simulink model "dinamica"  (R2022b)
settings: Solver=VariableStepAuto  StartTime=0.0  StopTime=4  RelTol=1e-5
undefined symbols (not defined in the file or in its folder): X, Y, Z
libraries: sm_lib x18, nesl_utility x13
settings Model: Creator=laurc  LastModifiedBy=laurc

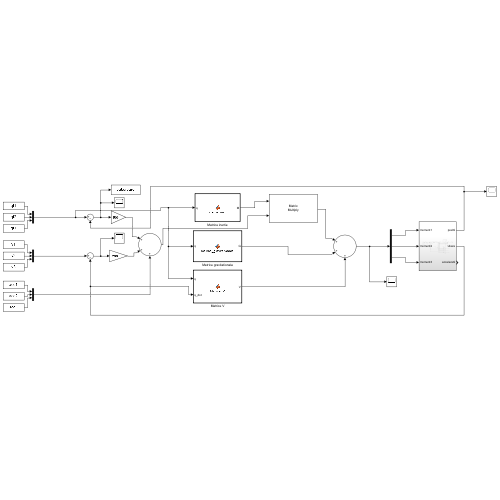
[thumbnail: Simulink's stored preview of the top-level diagram]
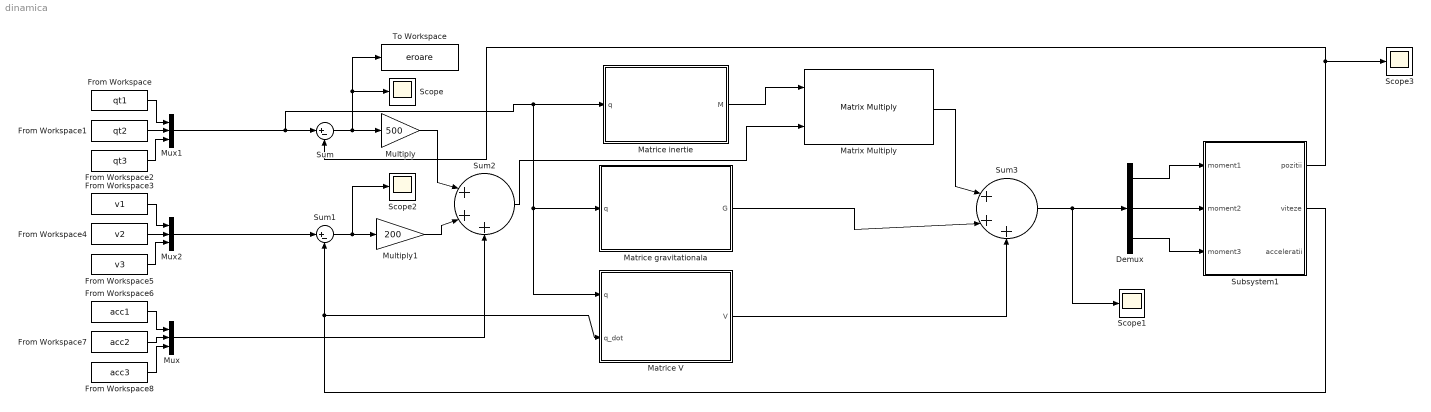
== system dinamica ==
  Demux : Demux  Outputs=3
  From Workspace : FromWorkspace  VariableName=qt1
  From Workspace1 : FromWorkspace  VariableName=qt2
  From Workspace2 : FromWorkspace  VariableName=qt3
  From Workspace3 : FromWorkspace  VariableName=v1
  From Workspace4 : FromWorkspace  VariableName=v2
  From Workspace5 : FromWorkspace  VariableName=v3
  From Workspace6 : FromWorkspace  VariableName=acc1
  From Workspace7 : FromWorkspace  VariableName=acc2
  From Workspace8 : FromWorkspace  VariableName=acc3
  Matrice V : MATLAB Function  TreatAsAtomicUnit=on
  Matrice gravitationala : MATLAB Function  TreatAsAtomicUnit=on
  Matrice inertie : MATLAB Function  TreatAsAtomicUnit=on
  Matrix Multiply : Product  Multiplication=Matrix(*)
  Multiply : Gain  Gain=500
  Multiply1 : Gain  Gain=200
  Mux : Mux  Inputs=3
  Mux1 : Mux  Inputs=3
  Mux2 : Mux  Inputs=3
  Scope{,1..3} (4 alike) : Scope
  Subsystem1 : Subsystem
  Sum : Sum  Inputs=|+-
  Sum1 : Sum  Inputs=|+-
  Sum2 : Sum  Inputs=|+++
  Sum3 : Sum  Inputs=|+++
  To Workspace : ToWorkspace  VariableName=eroare  SaveFormat=Timeseries  SampleTime=-1
  wires:
  Multiply1/1 -> Sum2/2
  Sum/1 -> Scope/1, To Workspace/1, Multiply/1
  From Workspace2/1 -> Mux1/3
  Sum1/1 -> Scope2/1, Multiply1/1
  From Workspace6/1 -> Mux/1
  Multiply/1 -> Sum2/1
  From Workspace7/1 -> Mux/2
  Mux2/1 -> Sum1/1
  Mux/1 -> Sum2/3
  From Workspace5/1 -> Mux2/3
  From Workspace8/1 -> Mux/3
  From Workspace/1 -> Mux1/1
  From Workspace3/1 -> Mux2/1
  From Workspace1/1 -> Mux1/2
  From Workspace4/1 -> Mux2/2
  Matrice inertie/1(M) -> Matrix Multiply/1
  Sum2/1 -> Matrix Multiply/2
  Matrix Multiply/1 -> Sum3/1
  Matrice gravitationala/1(G) -> Sum3/2
  Matrice V/1(V) -> Sum3/3
  Sum3/1 -> Scope1/1, Demux/1
  Demux/1 -> Subsystem1/1(moment1)
  Demux/2 -> Subsystem1/2(moment2)
  Demux/3 -> Subsystem1/3(moment3)
  Subsystem1/1(pozitii) -> Scope3/1, Sum/2
  Subsystem1/2(viteze) -> Sum1/2, Matrice V/2(q_dot)
  Mux1/1 -> Matrice V/1(q), Matrice gravitationala/1(q), Matrice inertie/1(q), Sum/1

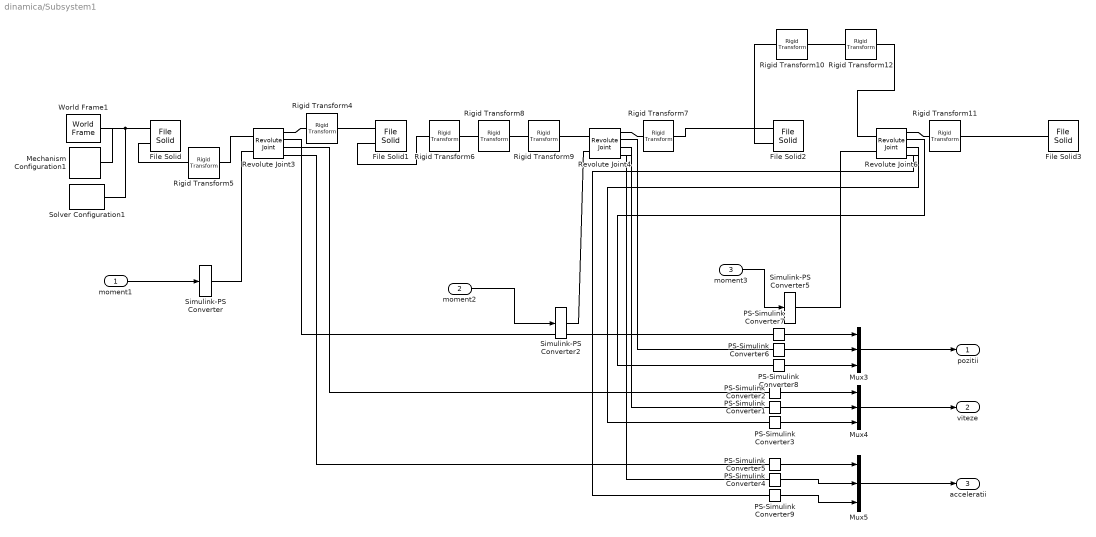
== system dinamica/Subsystem1 ==
  moment1 : Inport
  moment2 : Inport  Port=2
  moment3 : Inport  Port=3
  File Solid : sm_lib/Body Elements/File Solid  ExtGeomFileName=C:\Users\laurc\OneDrive\Desktop\robot puma nou\baza.stp  UnitType=FromFile  ExtGeomFileUnits=m  StepReaderType=HEX  ExportConvexHullGeometry=off  InertiaType=CalculateFromGeometry  Mass=1  MassUnits=kg  CenterOfMass=[0 0 0]  CenterOfMassUnits=m  MomentsOfInertia=[1 1 1]  MomentsOfInertiaUnits=kg*m^2  ProductsOfInertia=[0 0 0]  ProductsOfInertiaUnits=kg*m^2  BasedOnType=Density  Density=1000  DensityUnits=kg/m^3  DoExposeReferenceFrame=on  SerializedFrames=<Frames><Frame><Id>Frame1</Id><Value><Name>F1</Name><Origin><Source>ReferenceFrame</Source><FeatureName></FeatureName></Origin><PrimaryAxis><DefinedDirection>+Z</DefinedDirection><Source>ReferenceFrame</Source><SourceDirection>+Z</SourceDirection><FeatureName></FeatureName></PrimaryAxis><SecondaryAxis><DefinedDirection>+X</DefinedDirection><Source>ReferenceFrame</Source><SourceDirection>+X</SourceDirection><FeatureName></FeatureName></SecondaryAxis></Value></Frame><Frame><Id>Frame2</Id><Value><Name>F2</Name><Origin><Source>GeometricFeature</Source><FeatureName>circular curve 22</FeatureName></Origin><PrimaryAxis><DefinedDirection>+Z</DefinedDirection><Source>ReferenceFrame</Source><SourceDirection>+Z</SourceDirection><FeatureName></FeatureName></PrimaryAxis><SecondaryAxis><DefinedDirection>+X</DefinedDirection><Source>ReferenceFrame</Source><SourceDirection>+X</SourceDirection><FeatureName></FeatureName></SecondaryAxis></Value></Frame></Frames>  GraphicType=FromGeometry  MarkerShape=Sphere  MarkerSize=10  GraphicVisPropType=SimpleVisualProperties  GraphicDiffuseColor=[0.8 0.8 0.8]  GraphicSpecularColor=[0.5 0.5 0.5 1.0]  GraphicAmbientColor=[0.15 0.15 0.15 1.0]  GraphicEmissiveColor=[0.0 0.0 0.0 1.0]  GraphicShininess=75  GraphicOpacity=1.0
  File Solid1 : sm_lib/Body Elements/File Solid  ExtGeomFileName=C:\Users\laurc\OneDrive\Desktop\robot puma nou\brat1.stp  UnitType=FromFile  ExtGeomFileUnits=m  StepReaderType=HEX  ExportConvexHullGeometry=off  InertiaType=CalculateFromGeometry  Mass=1  MassUnits=kg  CenterOfMass=[0 0 0]  CenterOfMassUnits=m  MomentsOfInertia=[1 1 1]  MomentsOfInertiaUnits=kg*m^2  ProductsOfInertia=[0 0 0]  ProductsOfInertiaUnits=kg*m^2  BasedOnType=Density  Density=1000  DensityUnits=kg/m^3  DoExposeReferenceFrame=on  SerializedFrames=<Frames><Frame><Id>Frame1</Id><Value><Name>F1</Name><Origin><Source>GeometricFeature</Source><FeatureName>planar surface 1</FeatureName></Origin><PrimaryAxis><DefinedDirection>+Z</DefinedDirection><Source>ReferenceFrame</Source><SourceDirection>+Z</SourceDirection><FeatureName></FeatureName></PrimaryAxis><SecondaryAxis><DefinedDirection>+X</DefinedDirection><Source>ReferenceFrame</Source><SourceDirection>+X</SourceDirection><FeatureName></FeatureName></SecondaryAxis></Value></Frame><Frame><Id>Frame2</Id><Value><Name>F2</Name><Origin><Source>GeometricFeature</Source><FeatureName>planar surface 3</FeatureName></Origin><PrimaryAxis><DefinedDirection>+Z</DefinedDirection><Source>ReferenceFrame</Source><SourceDirection>+Z</SourceDirection><FeatureName></FeatureName></PrimaryAxis><SecondaryAxis><DefinedDirection>+X</DefinedDirection><Source>ReferenceFrame</Source><SourceDirection>+X</SourceDirection><FeatureName></FeatureName></SecondaryAxis></Value></Frame></Frames>  GraphicType=FromGeometry  MarkerShape=Sphere  MarkerSize=10  GraphicVisPropType=SimpleVisualProperties  GraphicDiffuseColor=[0.8 0.8 0.8]  GraphicSpecularColor=[0.5 0.5 0.5 1.0]  GraphicAmbientColor=[0.15 0.15 0.15 1.0]  GraphicEmissiveColor=[0.0 0.0 0.0 1.0]  GraphicShininess=75  GraphicOpacity=1.0
  File Solid2 : sm_lib/Body Elements/File Solid  ExtGeomFileName=C:\Users\laurc\OneDrive\Desktop\robot puma nou\brat2.stp  UnitType=FromFile  ExtGeomFileUnits=m  StepReaderType=HEX  ExportConvexHullGeometry=off  InertiaType=CalculateFromGeometry  Mass=1  MassUnits=kg  CenterOfMass=[0 0 0]  CenterOfMassUnits=m  MomentsOfInertia=[1 1 1]  MomentsOfInertiaUnits=kg*m^2  ProductsOfInertia=[0 0 0]  ProductsOfInertiaUnits=kg*m^2  BasedOnType=Density  Density=1000  DensityUnits=kg/m^3  DoExposeReferenceFrame=on  SerializedFrames=<Frames><Frame><Id>Frame1</Id><Value><Name>F1</Name><Origin><Source>GeometricFeature</Source><FeatureName>planar surface 2</FeatureName></Origin><PrimaryAxis><DefinedDirection>+X</DefinedDirection><Source>ReferenceFrame</Source><SourceDirection>+Z</SourceDirection><FeatureName></FeatureName></PrimaryAxis><SecondaryAxis><DefinedDirection>-Y</DefinedDirection><Source>ReferenceFrame</Source><SourceDirection>+X</SourceDirection><FeatureName></FeatureName></SecondaryAxis></Value></Frame><Frame><Id>Frame2</Id><Value><Name>F2</Name><Origin><Source>GeometricFeature</Source><FeatureName>planar surface 1</FeatureName></Origin><PrimaryAxis><DefinedDirection>+Z</DefinedDirection><Source>ReferenceFrame</Source><SourceDirection>+Z</SourceDirection><FeatureName></FeatureName></PrimaryAxis><SecondaryAxis><DefinedDirection>+X</DefinedDirection><Source>ReferenceFrame</Source><SourceDirection>+X</SourceDirection><FeatureName></FeatureName></SecondaryAxis></Value></Frame></Frames>  GraphicType=FromGeometry  MarkerShape=Sphere  MarkerSize=10  GraphicVisPropType=SimpleVisualProperties  GraphicDiffuseColor=[0.8 0.8 0.8]  GraphicSpecularColor=[0.5 0.5 0.5 1.0]  GraphicAmbientColor=[0.15 0.15 0.15 1.0]  GraphicEmissiveColor=[0.0 0.0 0.0 1.0]  GraphicShininess=75  GraphicOpacity=1.0
  File Solid3 : sm_lib/Body Elements/File Solid  ExtGeomFileName=C:\Users\laurc\OneDrive\Desktop\robot puma nou\efector.stp  UnitType=FromFile  ExtGeomFileUnits=m  StepReaderType=HEX  ExportConvexHullGeometry=off  InertiaType=CalculateFromGeometry  Mass=1  MassUnits=kg  CenterOfMass=[0 0 0]  CenterOfMassUnits=m  MomentsOfInertia=[1 1 1]  MomentsOfInertiaUnits=kg*m^2  ProductsOfInertia=[0 0 0]  ProductsOfInertiaUnits=kg*m^2  BasedOnType=Density  Density=1000  DensityUnits=kg/m^3  DoExposeReferenceFrame=on  SerializedFrames=<Frames><Frame><Id>Frame1</Id><Value><Name>F1</Name><Origin><Source>GeometricFeature</Source><FeatureName>planar surface 12</FeatureName></Origin><PrimaryAxis><DefinedDirection>+Z</DefinedDirection><Source>ReferenceFrame</Source><SourceDirection>+Z</SourceDirection><FeatureName></FeatureName></PrimaryAxis><SecondaryAxis><DefinedDirection>+X</DefinedDirection><Source>ReferenceFrame</Source><SourceDirection>+X</SourceDirection><FeatureName></FeatureName></SecondaryAxis></Value></Frame></Frames>  GraphicType=FromGeometry  MarkerShape=Sphere  MarkerSize=10  GraphicVisPropType=SimpleVisualProperties  GraphicDiffuseColor=[0.8 0.8 0.8]  GraphicSpecularColor=[0.5 0.5 0.5 1.0]  GraphicAmbientColor=[0.15 0.15 0.15 1.0]  GraphicEmissiveColor=[0.0 0.0 0.0 1.0]  GraphicShininess=75  GraphicOpacity=1.0
  Mechanism Configuration1 : sm_lib/Utilities/Mechanism Configuration  UniformGravity=Constant  GravityVector=[0 0 -9.80665]  GravityUnits=m/s^2  LinearizationDelta=0.001  JointModeTransitionNonlinearIterations=2
  Mux3 : Mux  Inputs=3
  Mux4 : Mux  Inputs=3
  Mux5 : Mux  Inputs=3
  PS-Simulink Converter{1..9} (9 alike) : nesl_utility/PS-Simulink Converter  PhysicalDomain=network_engine_domain  SubClassName=ps_output  LeftPortType=input  RightPortType=output  PseudoPeriodic=off  Frequencies=[]  VectorFormat=inherit  Unit=inherit  AffineConversion=off
  Revolute Joint3 : sm_lib/Joints/Revolute Joint  JointMode=Normal  SenseConstraintForce=off  SenseConstraintForceX=off  SenseConstraintForceY=off  SenseConstraintForceZ=off  SenseConstraintTorque=off  SenseConstraintTorqueX=off  SenseConstraintTorqueY=off  SenseConstraintTorqueZ=off  SenseTotalForce=off  SenseTotalForceX=off  SenseTotalForceY=off  SenseTotalForceZ=off  SenseTotalTorque=off  SenseTotalTorqueX=off  SenseTotalTorqueY=off  SenseTotalTorqueZ=off  CompositeWrenchDir=FollowerOnBase  CompositeWrenchFrame=BaseFrame  EquilibriumPosition=0  EquilibriumPositionUnits=deg  SpringStiffness=0  SpringStiffnessUnits=N*m/deg  DampingCoefficient=0  DampingCoefficientUnits=N*m/(deg/s)  TorqueActuationMode=ComputedTorque  MotionActuationMode=InputMotion  SensePosition=on  SenseVelocity=on  SenseAcceleration=on  SenseTorqueForce=off  SenseLowerLimitTorqueForce=off  SenseUpperLimitTorqueForce=off  LowerLimitSpecify=off  LowerLimitBound=-90  LowerLimitBoundUnits=deg  LowerLimitStiffness=1e4  LowerLimitStiffnessUnits=N*m/deg  LowerLimitDamping=10  LowerLimitDampingUnits=N*m/(deg/s)  LowerLimitTransitionRegionWidth=0.1  LowerLimitTransitionRegionWidthUnits=deg  UpperLimitSpecify=off  UpperLimitBound=90  UpperLimitBoundUnits=deg  UpperLimitStiffness=1e4  UpperLimitStiffnessUnits=N*m/deg  UpperLimitDamping=10  UpperLimitDampingUnits=N*m/(deg/s)  UpperLimitTransitionRegionWidth=0.1  UpperLimitTransitionRegionWidthUnits=deg  PositionTargetSpecify=off  PositionTargetPriority=High  PositionTargetValue=0  PositionTargetValueUnits=deg  VelocityTargetSpecify=off  VelocityTargetPriority=High  VelocityTargetValue=0  VelocityTargetValueUnits=deg/s
  Revolute Joint4 : sm_lib/Joints/Revolute Joint  JointMode=Normal  SenseConstraintForce=off  SenseConstraintForceX=off  SenseConstraintForceY=off  SenseConstraintForceZ=off  SenseConstraintTorque=off  SenseConstraintTorqueX=off  SenseConstraintTorqueY=off  SenseConstraintTorqueZ=off  SenseTotalForce=off  SenseTotalForceX=off  SenseTotalForceY=off  SenseTotalForceZ=off  SenseTotalTorque=off  SenseTotalTorqueX=off  SenseTotalTorqueY=off  SenseTotalTorqueZ=off  CompositeWrenchDir=FollowerOnBase  CompositeWrenchFrame=BaseFrame  EquilibriumPosition=0  EquilibriumPositionUnits=deg  SpringStiffness=0  SpringStiffnessUnits=N*m/deg  DampingCoefficient=0  DampingCoefficientUnits=N*m/(deg/s)  TorqueActuationMode=ComputedTorque  MotionActuationMode=InputMotion  SensePosition=on  SenseVelocity=on  SenseAcceleration=on  SenseTorqueForce=off  SenseLowerLimitTorqueForce=off  SenseUpperLimitTorqueForce=off  LowerLimitSpecify=off  LowerLimitBound=-90  LowerLimitBoundUnits=deg  LowerLimitStiffness=1e4  LowerLimitStiffnessUnits=N*m/deg  LowerLimitDamping=10  LowerLimitDampingUnits=N*m/(deg/s)  LowerLimitTransitionRegionWidth=0.1  LowerLimitTransitionRegionWidthUnits=deg  UpperLimitSpecify=off  UpperLimitBound=90  UpperLimitBoundUnits=deg  UpperLimitStiffness=1e4  UpperLimitStiffnessUnits=N*m/deg  UpperLimitDamping=10  UpperLimitDampingUnits=N*m/(deg/s)  UpperLimitTransitionRegionWidth=0.1  UpperLimitTransitionRegionWidthUnits=deg  PositionTargetSpecify=off  PositionTargetPriority=High  PositionTargetValue=0  PositionTargetValueUnits=deg  VelocityTargetSpecify=off  VelocityTargetPriority=High  VelocityTargetValue=0  VelocityTargetValueUnits=deg/s
  Revolute Joint6 : sm_lib/Joints/Revolute Joint  JointMode=Normal  SenseConstraintForce=off  SenseConstraintForceX=off  SenseConstraintForceY=off  SenseConstraintForceZ=off  SenseConstraintTorque=off  SenseConstraintTorqueX=off  SenseConstraintTorqueY=off  SenseConstraintTorqueZ=off  SenseTotalForce=off  SenseTotalForceX=off  SenseTotalForceY=off  SenseTotalForceZ=off  SenseTotalTorque=off  SenseTotalTorqueX=off  SenseTotalTorqueY=off  SenseTotalTorqueZ=off  CompositeWrenchDir=FollowerOnBase  CompositeWrenchFrame=BaseFrame  EquilibriumPosition=0  EquilibriumPositionUnits=deg  SpringStiffness=0  SpringStiffnessUnits=N*m/deg  DampingCoefficient=0  DampingCoefficientUnits=N*m/(deg/s)  TorqueActuationMode=ComputedTorque  MotionActuationMode=InputMotion  SensePosition=on  SenseVelocity=on  SenseAcceleration=on  SenseTorqueForce=off  SenseLowerLimitTorqueForce=off  SenseUpperLimitTorqueForce=off  LowerLimitSpecify=off  LowerLimitBound=-90  LowerLimitBoundUnits=deg  LowerLimitStiffness=1e4  LowerLimitStiffnessUnits=N*m/deg  LowerLimitDamping=10  LowerLimitDampingUnits=N*m/(deg/s)  LowerLimitTransitionRegionWidth=0.1  LowerLimitTransitionRegionWidthUnits=deg  UpperLimitSpecify=off  UpperLimitBound=90  UpperLimitBoundUnits=deg  UpperLimitStiffness=1e4  UpperLimitStiffnessUnits=N*m/deg  UpperLimitDamping=10  UpperLimitDampingUnits=N*m/(deg/s)  UpperLimitTransitionRegionWidth=0.1  UpperLimitTransitionRegionWidthUnits=deg  PositionTargetSpecify=off  PositionTargetPriority=High  PositionTargetValue=0  PositionTargetValueUnits=deg  VelocityTargetSpecify=off  VelocityTargetPriority=High  VelocityTargetValue=0  VelocityTargetValueUnits=deg/s
  Rigid Transform10 : sm_lib/Frames and Transforms/Rigid Transform  TranslationMethod=Cartesian  TranslationStandardOffset=0  TranslationLengthUnit=mm  TranslationStandardAxis=+Z  TranslationCartesianOffset=[0 -0 -60]  TranslationROffset=0  TranslationROffsetUnits=m  TranslationZOffset=0  TranslationZOffsetUnits=m  TranslationThetaOffset=0  TranslationThetaOffsetUnits=deg  RotationMethod=StandardAxis  RotationAngleUnits=deg  RotationStandardAxis=-Y  RotationAngle=90  RotationArbitraryAxis=[0 0 1]  FollAlignAxisA=+X  BaseAlignAxisA=+Y  FollAlignAxisB=+Y  BaseAlignAxisB=+Z  RotationSequenceAxes=FollowerAxes  RotationSequence=XYX  RotationSequenceAngles=[0 0 0]  RotationSequenceAnglesUnits=deg  RotationMatrix=[1 0 0; 0 1 0; 0 0 1]  Quaternion=[1 0 0 0]
  Rigid Transform11 : sm_lib/Frames and Transforms/Rigid Transform  TranslationMethod=Cartesian  TranslationStandardOffset=0  TranslationLengthUnit=mm  TranslationStandardAxis=+Z  TranslationCartesianOffset=[0 0 0]  TranslationROffset=0  TranslationROffsetUnits=m  TranslationZOffset=0  TranslationZOffsetUnits=m  TranslationThetaOffset=0  TranslationThetaOffsetUnits=deg  RotationMethod=StandardAxis  RotationAngleUnits=deg  RotationStandardAxis=+Y  RotationAngle=90  RotationArbitraryAxis=[0 0 1]  FollAlignAxisA=+X  BaseAlignAxisA=+Y  FollAlignAxisB=+Y  BaseAlignAxisB=+Z  RotationSequenceAxes=FollowerAxes  RotationSequence=XYX  RotationSequenceAngles=[0 0 0]  RotationSequenceAnglesUnits=deg  RotationMatrix=[1 0 0; 0 1 0; 0 0 1]  Quaternion=[1 0 0 0]
  Rigid Transform12 : sm_lib/Frames and Transforms/Rigid Transform  TranslationMethod=Cartesian  TranslationStandardOffset=0  TranslationLengthUnit=mm  TranslationStandardAxis=+Z  TranslationCartesianOffset=[0 0 0]  TranslationROffset=0  TranslationROffsetUnits=m  TranslationZOffset=0  TranslationZOffsetUnits=m  TranslationThetaOffset=0  TranslationThetaOffsetUnits=deg  RotationMethod=StandardAxis  RotationAngleUnits=deg  RotationStandardAxis=-Y  RotationAngle=90  RotationArbitraryAxis=[0 0 1]  FollAlignAxisA=+X  BaseAlignAxisA=+Y  FollAlignAxisB=+Y  BaseAlignAxisB=+Z  RotationSequenceAxes=FollowerAxes  RotationSequence=XYX  RotationSequenceAngles=[0 0 0]  RotationSequenceAnglesUnits=deg  RotationMatrix=[1 0 0; 0 1 0; 0 0 1]  Quaternion=[1 0 0 0]
  Rigid Transform4 : sm_lib/Frames and Transforms/Rigid Transform  TranslationMethod=None  TranslationStandardOffset=0  TranslationLengthUnit=mm  TranslationStandardAxis=+Z  TranslationCartesianOffset=0  TranslationROffset=0  TranslationROffsetUnits=m  TranslationZOffset=0  TranslationZOffsetUnits=m  TranslationThetaOffset=0  TranslationThetaOffsetUnits=deg  RotationMethod=StandardAxis  RotationAngleUnits=deg  RotationStandardAxis=-Y  RotationAngle=90  RotationArbitraryAxis=[0 0 1]  FollAlignAxisA=+X  BaseAlignAxisA=+Y  FollAlignAxisB=+Y  BaseAlignAxisB=+Z  RotationSequenceAxes=FollowerAxes  RotationSequence=XYX  RotationSequenceAngles=[0 0 0]  RotationSequenceAnglesUnits=deg  RotationMatrix=[1 0 0; 0 1 0; 0 0 1]  Quaternion=[1 0 0 0]
  Rigid Transform5 : sm_lib/Frames and Transforms/Rigid Transform  TranslationMethod=Cartesian  TranslationStandardOffset=0  TranslationLengthUnit=mm  TranslationStandardAxis=+Y  TranslationCartesianOffset=[0 31 0]  TranslationROffset=0  TranslationROffsetUnits=m  TranslationZOffset=0  TranslationZOffsetUnits=m  TranslationThetaOffset=0  TranslationThetaOffsetUnits=deg  RotationMethod=StandardAxis  RotationAngleUnits=deg  RotationStandardAxis=+X  RotationAngle=90  RotationArbitraryAxis=[0 0 1]  FollAlignAxisA=+X  BaseAlignAxisA=+Y  FollAlignAxisB=+Y  BaseAlignAxisB=+Z  RotationSequenceAxes=FollowerAxes  RotationSequence=XYX  RotationSequenceAngles=[0 0 0]  RotationSequenceAnglesUnits=deg  RotationMatrix=[1 0 0; 0 1 0; 0 0 1]  Quaternion=[1 0 0 0]
  Rigid Transform6 : sm_lib/Frames and Transforms/Rigid Transform  TranslationMethod=Cartesian  TranslationStandardOffset=0  TranslationLengthUnit=mm  TranslationStandardAxis=+Z  TranslationCartesianOffset=[0 30 0]  TranslationROffset=0  TranslationROffsetUnits=m  TranslationZOffset=0  TranslationZOffsetUnits=m  TranslationThetaOffset=0  TranslationThetaOffsetUnits=deg  RotationMethod=StandardAxis  RotationAngleUnits=deg  RotationStandardAxis=-X  RotationAngle=90  RotationArbitraryAxis=[0 0 1]  FollAlignAxisA=+X  BaseAlignAxisA=+Y  FollAlignAxisB=+Y  BaseAlignAxisB=+Z  RotationSequenceAxes=FollowerAxes  RotationSequence=XYX  RotationSequenceAngles=[0 0 0]  RotationSequenceAnglesUnits=deg  RotationMatrix=[1 0 0; 0 1 0; 0 0 1]  Quaternion=[1 0 0 0]
  Rigid Transform7 : sm_lib/Frames and Transforms/Rigid Transform  TranslationMethod=None  TranslationStandardOffset=0  TranslationLengthUnit=mm  TranslationStandardAxis=+Z  TranslationCartesianOffset=[0 294.5 141.5]  TranslationROffset=0  TranslationROffsetUnits=m  TranslationZOffset=0  TranslationZOffsetUnits=m  TranslationThetaOffset=0  TranslationThetaOffsetUnits=deg  RotationMethod=StandardAxis  RotationAngleUnits=deg  RotationStandardAxis=+Y  RotationAngle=90  RotationArbitraryAxis=[0 0 1]  FollAlignAxisA=+X  BaseAlignAxisA=+Y  FollAlignAxisB=+Y  BaseAlignAxisB=+Z  RotationSequenceAxes=FollowerAxes  RotationSequence=XYX  RotationSequenceAngles=[0 0 0]  RotationSequenceAnglesUnits=deg  RotationMatrix=[1 0 0; 0 1 0; 0 0 1]  Quaternion=[1 0 0 0]
  Rigid Transform8 : sm_lib/Frames and Transforms/Rigid Transform  TranslationMethod=Cartesian  TranslationStandardOffset=0  TranslationLengthUnit=mm  TranslationStandardAxis=+Z  TranslationCartesianOffset=[0 0 30]  TranslationROffset=0  TranslationROffsetUnits=m  TranslationZOffset=0  TranslationZOffsetUnits=m  TranslationThetaOffset=0  TranslationThetaOffsetUnits=deg  RotationMethod=StandardAxis  RotationAngleUnits=deg  RotationStandardAxis=-Y  RotationAngle=90  RotationArbitraryAxis=[0 0 1]  FollAlignAxisA=+X  BaseAlignAxisA=+Y  FollAlignAxisB=+Y  BaseAlignAxisB=+Z  RotationSequenceAxes=FollowerAxes  RotationSequence=XYX  RotationSequenceAngles=[0 0 0]  RotationSequenceAnglesUnits=deg  RotationMatrix=[1 0 0; 0 1 0; 0 0 1]  Quaternion=[1 0 0 0]
  Rigid Transform9 : sm_lib/Frames and Transforms/Rigid Transform  TranslationMethod=None  TranslationStandardOffset=0  TranslationLengthUnit=mm  TranslationStandardAxis=+Z  TranslationCartesianOffset=[0 294.5 141.5]  TranslationROffset=0  TranslationROffsetUnits=m  TranslationZOffset=0  TranslationZOffsetUnits=m  TranslationThetaOffset=0  TranslationThetaOffsetUnits=deg  RotationMethod=StandardAxis  RotationAngleUnits=deg  RotationStandardAxis=+Y  RotationAngle=90  RotationArbitraryAxis=[0 0 1]  FollAlignAxisA=+X  BaseAlignAxisA=+Y  FollAlignAxisB=+Y  BaseAlignAxisB=+Z  RotationSequenceAxes=FollowerAxes  RotationSequence=XYX  RotationSequenceAngles=[0 0 0]  RotationSequenceAnglesUnits=deg  RotationMatrix=[1 0 0; 0 1 0; 0 0 1]  Quaternion=[1 0 0 0]
  Simulink-PS Converter : nesl_utility/Simulink-PS Converter  PhysicalDomain=network_engine_domain  SubClassName=ps_input  LeftPortType=input  RightPortType=output  PseudoPeriodic=off  Frequencies=[]  NoiseDistribution=none  NoiseParameters=[]  Unit=1  AffineConversion=off  FilteringAndDerivatives=filter  SimscapeFilterOrder=2  InputFilterTimeConstant=0.001  UdotUserProvided=0
  Simulink-PS Converter2 : nesl_utility/Simulink-PS Converter  PhysicalDomain=network_engine_domain  SubClassName=ps_input  LeftPortType=input  RightPortType=output  PseudoPeriodic=off  Frequencies=[]  NoiseDistribution=none  NoiseParameters=[]  Unit=1  AffineConversion=off  FilteringAndDerivatives=filter  SimscapeFilterOrder=2  InputFilterTimeConstant=0.001  UdotUserProvided=0
  Simulink-PS Converter5 : nesl_utility/Simulink-PS Converter  PhysicalDomain=network_engine_domain  SubClassName=ps_input  LeftPortType=input  RightPortType=output  PseudoPeriodic=off  Frequencies=[]  NoiseDistribution=none  NoiseParameters=[]  Unit=1  AffineConversion=off  FilteringAndDerivatives=filter  SimscapeFilterOrder=2  InputFilterTimeConstant=0.001  UdotUserProvided=0
  Solver Configuration1 : nesl_utility/Solver Configuration  PhysicalDomain=network_engine_domain  SubClassName=solver  LeftPortType=input  RightPortType=generic  Tones=[]  Harmonics=[]  SimulateNoise=off  Profile=off  UseLocalSampling=off  EnableSwitchedLinearOptims=on  FrequencyDomain=off  UseCCode=off  RelTol=0.001  AbsTol=0.001  MinStep=1e-09  ToWorkspace=off  RevertToSquareIcSolve=off  NumHomotopyIterations=100  PhasorMode=off  PhasorModeNumHarmonics=1  ConsistencySolver=NEWTON_XTOL_AFTER_FTOL  IndexReductionMethod=DerivativeReplacement  DoDC=off  ResidualTolerance=1e-09  ConsistencyTolSource=GLOBAL  ConsistencyAbsTol=0.001  ConsistencyRelTol=0.001  ConsistencyTolFactor=0.001  UseLocalSolver=off  LocalSolverChoice=NE_BACKWARD_EULER_ADVANCER  ResolveIndetEquations=on  FunctionEvalNumThread=1  LocalSolverSampleTime=0.001  DoFixedCost=off  MaxNonlinIter=3  MaxModeIter=2  ComputeImpulses=off  ImpulseIterations=2  LinearAlgebra=auto  LinearAlgebraNumThread=0  EquationFormulation=NE_TIME_EF  DelaysMemoryBudget=1024  AutomaticFiltering=on  FilteringTimeConstant=0.001  PartitionStorageMethod=AS_NEEDED  PartitionMemoryBudget=1024  PartitionMethod=ROBUST
  World Frame1 : sm_lib/Frames and Transforms/World Frame
  pozitii : Outport
  viteze : Outport  Port=2
  acceleratii : Outport  Port=3
  wires:
  Mux4/1 -> viteze/1
  moment2/1 -> Simulink-PS Converter2/1
  moment3/1 -> Simulink-PS Converter5/1
  PS-Simulink Converter4/1 -> Mux5/2
  Mux5/1 -> acceleratii/1
  PS-Simulink Converter7/1 -> Mux3/1
  PS-Simulink Converter2/1 -> Mux4/1
  PS-Simulink Converter8/1 -> Mux3/3
  PS-Simulink Converter1/1 -> Mux4/2
  Mux3/1 -> pozitii/1
  PS-Simulink Converter9/1 -> Mux5/3
  PS-Simulink Converter3/1 -> Mux4/3
  PS-Simulink Converter5/1 -> Mux5/1
  moment1/1 -> Simulink-PS Converter/1
  PS-Simulink Converter6/1 -> Mux3/2
  connections:
  Revolute Joint4/RConn3 -- PS-Simulink Converter1/LConn1
  Revolute Joint4/RConn2 -- PS-Simulink Converter6/LConn1
  Rigid Transform7/RConn1 -- File Solid2/LConn1
  Rigid Transform6/RConn1 -- Rigid Transform8/LConn1
  Revolute Joint6/RConn3 -- PS-Simulink Converter3/LConn1
  Revolute Joint6/RConn1 -- Rigid Transform11/LConn1
  Revolute Joint4/RConn4 -- PS-Simulink Converter4/LConn1
  Revolute Joint3/RConn3 -- PS-Simulink Converter2/LConn1
  Revolute Joint4/RConn1 -- Rigid Transform7/LConn1
  File Solid/LConn1 -- Solver Configuration1/RConn1 -- World Frame1/RConn1 -- Mechanism Configuration1/RConn1
  Rigid Transform10/LConn1 -- File Solid2/LConn2
  Rigid Transform10/RConn1 -- Rigid Transform12/LConn1
  File Solid1/LConn2 -- Rigid Transform6/LConn1
  Revolute Joint4/LConn1 -- Rigid Transform9/RConn1
  Revolute Joint3/LConn1 -- Rigid Transform5/RConn1
  File Solid3/LConn1 -- Rigid Transform11/RConn1
  Rigid Transform4/RConn1 -- File Solid1/LConn1
  Revolute Joint6/LConn1 -- Rigid Transform12/RConn1
  Revolute Joint3/RConn1 -- Rigid Transform4/LConn1
  File Solid/LConn2 -- Rigid Transform5/LConn1
  Rigid Transform8/RConn1 -- Rigid Transform9/LConn1
  Revolute Joint6/RConn2 -- PS-Simulink Converter8/LConn1
  Revolute Joint6/RConn4 -- PS-Simulink Converter9/LConn1
  Revolute Joint3/RConn4 -- PS-Simulink Converter5/LConn1
  Revolute Joint3/RConn2 -- PS-Simulink Converter7/LConn1
  Simulink-PS Converter/RConn1 -- Revolute Joint3/LConn2
  Simulink-PS Converter2/RConn1 -- Revolute Joint4/LConn2
  Simulink-PS Converter5/RConn1 -- Revolute Joint6/LConn2

== matlab function dinamica/Matrice inertie ==
  data: q input; M output
function M = inertia_mat(q)

%xc=centre de masa 
%m-masa
%ixx=matricea de inertie  
%x2 y2 disntanta intre cuple

%Inlocuite
xc_1 = -0.36; yc_1 = 70.689; zc_1 = 0;
Ixx_1 = 0.0007006; Iyy_1 = 0.0001766; Izz_1 = 0.0006981; m_1 = 0.381;

xc_2 = 0; yc_2 = 127.75; zc_2 = 0;
Ixx_2 = 0.003; Iyy_2 = 0.0002608; Izz_2 = 0.003; m_2 = 0.618;

xc_3 = -0.15; yc_3 = 124.842; zc_3 = 0;
Ixx_3 = 0.004; Iyy_3 = 0.000264; Izz_3 = 0.004; m_3 = 0.633;

x_3 = 0; y_3 =-185.3; z_3 =171.5;
x_2 = 0; y_2 =30; z_2 =121.5;

m_11 = m_1 * (xc_1^2 + yc_1^2) + m_2 * ((xc_2*cos(q(2,:)) + zc_2 * sin(q(2,:)) + x_2)^2 + (yc_2 + y_2)^2) + m_3 * ((xc_3*cos(q(2,:) + q(3,:)) + zc_3 * sin(q(2,:) + q(3,:)) + x_3*cos(q(2,:)) + z_3 * sin(q(2,:)) + x_2)^2 + (yc_3 + y_3 + y_2)^2) + Izz_1 + Izz_2 + Izz_3;
m_12 = -m_2 * (yc_2 + y_2) * (-xc_2 * sin(q(2,:)) + zc_2 * cos(q(2,:))) - m_3 * (yc_3 + y_3 + y_2) * (-xc_3 * sin(q(2,:) + q(3,:)) + zc_3 * cos(q(2,:) + q(3,:)) -x_3 * sin(q(2,:)) + z_3 * cos(q(2,:)));
m_13 = - m_3 * (yc_3 + y_3 + y_2) * (-xc_3 * sin(q(2,:) + q(3,:)) + zc_3 * cos(q(2,:) + q(3,:)));

m_21 = m_12;
m_22 = m_2 * ((-xc_2 * sin(q(2,:)) + zc_2 * cos(q(2,:)))^2 + (xc_2*cos(q(2,:)) + zc_2 * sin(q(2,:)))^2) + m_3 * ((-xc_3 * sin(q(2,:) + q(3,:)) + zc_3 * cos(q(2,:) + q(3,:)) -x_3 * sin(q(2,:)) + z_3 * cos(q(2,:))) ^2 + (xc_3*cos(q(2,:) + q(3,:)) + zc_3 * sin(q(2,:) + q(3,:)) + x_3*cos(q(2,:)) + z_3 * sin(q(2,:)))^2) + (Ixx_2 + Ixx_3) * sin(q(1,:))^2 + (Iyy_2 + Iyy_3) * cos(q(1,:))^2;
m_23 = m_3 * ( (-xc_3 * sin(q(2,:) + q(3,:)) + zc_3 * cos(q(2,:) + q(3,:)) -x_3 * sin(q(2,:)) + z_3 * cos(q(2,:))) * (-xc_3 * sin(q(2,:) + q(3,:)) + zc_3 * cos(q(2,:) + q(3,:))) + (xc_3*cos(q(2,:) + q(3,:)) + zc_3 * sin(q(2,:) + q(3,:)) + x_3*cos(q(2,:)) + z_3 * sin(q(2,:))) * (xc_3*cos(q(2,:) + q(3,:)) + zc_3 * sin(q(2,:) + q(3,:)))) + Ixx_3 * sin(q(1,:))^2 + Iyy_3 * cos(q(1,:))^2;

m_31 = m_13 ;
m_32 = m_23;
m_33 = m_3 * (xc_3 ^ 2 + zc_3 ^2) + Ixx_3 * sin(q(1,:))^2 + Iyy_3 * cos(q(1,:))^2;

M=[m_11, m_12, m_13;
    m_21, m_22, m_23;
    m_31, m_32, m_33;];

== matlab function dinamica/Matrice V ==
  data: q input; V output; q_dot input
function V = Matrice_V(q,q_dot)

xc_1 = -0.36; yc_1 = 70.689; zc_1 = 0;
Ixx_1 = 0.0007006; Iyy_1 = 0.0001766; Izz_1 = 0.0006981; m_1 = 0.381;

xc_2 = 0; yc_2 = 127.75; zc_2 = 0;
Ixx_2 = 0.003; Iyy_2 = 0.0002608; Izz_2 = 0.003; m_2 = 0.618;

xc_3 = -0.15; yc_3 = 124.842; zc_3 = 0;
Ixx_3 = 0.004; Iyy_3 = 0.000264; Izz_3 = 0.004; m_3 = 0.633;

x_3 = 0; y_3 =-185.3; z_3 =171.5;
x_2 = 0; y_2 =30; z_2 =121.5;


b_111=0;
b_122=m_2*(xc_2*cos(q(2,:)) + zc_2 * sin(q(2,:)))*(yc_2+y_2)+m_3*(xc_3*cos(q(2,:) + q(3,:)) + zc_3 * sin(q(2,:) + q(3,:)) + x_3*cos(q(2,:)) + z_3 * sin(q(2,:)))*(yc_3 + y_3 + y_2)-((Ixx_2 + Ixx_3) * sin(q(1,:)) * cos(q(1,:)) - (Iyy_2 + Iyy_3) * cos(q(1,:)) * sin(q(1,:)));
b_133=m_3*(yc_3+y_3+y_2)*(xc_3*cos(q(2,:) + q(3,:)) + zc_3 * sin(q(2,:) + q(3,:))-(Ixx_3-Iyy_3)*cos(q(1,:))*sin(q(1,:)));

b_211=-m_2*(xc_2*cos(q(2,:)) + zc_2 * sin(q(2,:)) + x_2)*(-xc_2 * sin(q(2,:)) + zc_2 * cos(q(2,:)))-m_3*(xc_3*cos(q(2,:) + q(3,:)) + zc_3 * sin(q(2,:) + q(3,:)) + x_3*cos(q(2,:)) + z_3 * sin(q(2,:)) + x_2)*(-xc_3 * sin(q(2,:) + q(3,:)) + zc_3 * cos(q(2,:) + q(3,:)) -x_3 * sin(q(2,:)) + z_3 * cos(q(2,:)));
b_222=0;
b_233=-m_3*((xc_3*cos(q(2,:) + q(3,:)) + zc_3 * sin(q(2,:) + q(3,:)))*(-xc_3 * sin(q(2,:) + q(3,:)) + zc_3 * cos(q(2,:) + q(3,:)))+(-xc_3 * sin(q(2,:) + q(3,:)) + zc_3 * cos(q(2,:) + q(3,:))-x_3 * sin(q(2,:)) + z_3 * cos(q(2,:)))*(xc_3*cos(q(2,:) + q(3,:)) + zc_3 * sin(q(2,:) + q(3,:))));

b_311=-m_3*(-xc_3*sin(q(2,:)+q(3,:)) + zc_3*cos(q(2,:)+q(3,:)))*(xc_3*cos(q(2,:)+q(3,:))+zc_3*sin(q(2,:)+q(3,:))+x_3*cos(q(2,:))+z_3*sin(q(2,:))+x_2);
b_322=-m_3*(-(-xc_3 * sin(q(2,:) + q(3,:)) + zc_3 * cos(q(2,:) + q(3,:))-x_3 * sin(q(2,:)) + z_3 * cos(q(2,:)))*(xc_3*cos(q(2,:) + q(3,:)) + zc_3 * sin(q(2,:) + q(3,:))) + (xc_3*cos(q(2,:)+q(3,:))+zc_3*sin(q(2,:)+q(3,:))+x_3*cos(q(2,:))+z_3*sin(q(2,:)))*(-xc_3 * sin(q(2,:) + q(3,:)) + zc_3 * cos(q(2,:) + q(3,:))));
b_333=0;

C=[b_111, b_122, b_133;
   b_211, b_222, b_233;
   b_311, b_322, b_333];

b_112 = -2 * b_211;
b_113 = -2 * b_311;
b_123 = 2 * (m_3 * (yc_3 + y_3 + y_2) * (-xc_3 * cos(q(2,:) + q(3,:)) + zc_3 *  sin(q(2,:) + q(3,:))) - (Ixx_3 - Iyy_3)*cos(q(1,:))*sin(q(1,:)));

b_212 = 2 * (Ixx_3 + Ixx_2 - Iyy_3 - Iyy_2)*cos(q(1,:))*sin(q(1,:));
b_213 = 2 * (Ixx_3 - Iyy_3)*cos(q(1,:))*sin(q(1,:));
b_223 = 2 * m_3 * (-(-xc_3 * sin(q(2,:) + q(3,:)) + zc_3 * cos(q(2,:) + q(3,:)) -x_3 * sin(q(2,:)) + z_3 * cos(q(2,:)))*(xc_3*cos(q(2,:) + q(3,:)) + zc_3 * sin(q(2,:) + q(3,:))) + (xc_3*cos(q(2,:) + q(3,:)) + zc_3 * sin(q(2,:) + q(3,:)) + x_3*cos(q(2,:)) + z_3 * sin(q(2,:)))*(-xc_3 * sin(q(2,:) + q(3,:)) + zc_3 * cos(q(2,:) + q(3,:))));

b_312 = b_213;
b_313 = b_213;
b_323 = 0;

B = [b_112,b_113,b_123;
    b_212, b_213, b_223;
    b_312, b_313, b_323;];


V = C * [q_dot(1,:)^2; q_dot(2,:)^2; q_dot(3,:)^2] + B * [q_dot(1,:)*q_dot(2,:);q_dot(1,:)*q_dot(3,:);q_dot(2,:)*q_dot(3,:);];

== matlab function dinamica/Matrice gravitationala ==
  data: q input; G output
function G = matrice_gravitationala(q)
g=9.81;
xc_1 = -0.36; yc_1 = 70.689; zc_1 = 0;
Ixx_1 = 0.0007006; Iyy_1 = 0.0001766; Izz_1 = 0.0006981; m_1 = 0.381;

xc_2 = 0; yc_2 = 127.75; zc_2 = 0;
Ixx_2 = 0.003; Iyy_2 = 0.0002608; Izz_2 = 0.003; m_2 = 0.618;

xc_3 = -0.15; yc_3 = 124.842; zc_3 = 0;
Ixx_3 = 0.004; Iyy_3 = 0.000264; Izz_3 = 0.004; m_3 = 0.633;

x_3 = 0; y_3 =-185.3; z_3 =171.5;
x_2 = 0; y_2 =30; z_2 =121.5;

g_1=0;
g_2=-m_2*(xc_2*cos(q(2,:))+zc_2*sin(q(2,:)))*g-m_3*(xc_3*cos(q(2,:)+q(3,:))+zc_3*sin(q(2,:)+q(3,:))+x_3*cos(q(2,:))+z_3*sin(q(2,:)))*g;
g_3=-m_3*(xc_3*cos(q(2,:)+q(3,:))+zc_3*sin(q(2,:)+q(3,:)))*g;
G=[g_1;g_2;g_3];
